simulink model "ThreeLevelANPC_16_11_22_cmv"  (R2021a)
settings: Solver=FixedStepAuto  StartTime=0.0  StopTime=0.1  RelTol=1e-3
model workspace (MAT data in the model file):
  Cdc = 0.000333333333333
  Cf = 9.4e-06
  Ctrap1 = 6e-06
  Ctrap2 = 4e-06
  DPWMGain = 1.04
  IdRef = 127
  IqRef = 0
  Lc = 0.0005
  Lf1 = 0.00015
  Lf2 = 4e-05
  Ltotal = 0.00019
  RLf1 = 0.003
  Rtrap = 0.1
  RtrapP1 = 100
  RtrapP2 = 100
  Ts = 1e-07
  Vdc = 1400
  VppRMS = 800
  fgrid = 50
  fs = 32000
  ki = 1
  ki_th = 600
  kidc = 0.1
  kidc_th = 0.05
  kp = 1
  kp_th = 600
  kpdc = 0.00166666666667
  kpdc_th = 0.05
  offset = -15
  third = 0.16
undefined symbols (not defined in the file or in its folder): C, DiscIntNeverNeededParam
libraries: spsSeriesRLCBranchLib x18, spsCurrentMeasurementLib x16, spsIGBTDiodeLib x12, spsParallelRLCBranchLib x12, spsVoltageMeasurementLib x8, spsMosfetLib x6, simulink x3, dspobslib x3, spsGroundLib x2, spsabctodq0Lib x2, eeGeneralControl x2, spsDCVoltageSourceLib x1
settings Model: OrderedModelArguments=off  Creator=ayberk.filik  LastModifiedBy=enes_
settings DataIOCC: ReturnWorkspaceOutputs=off

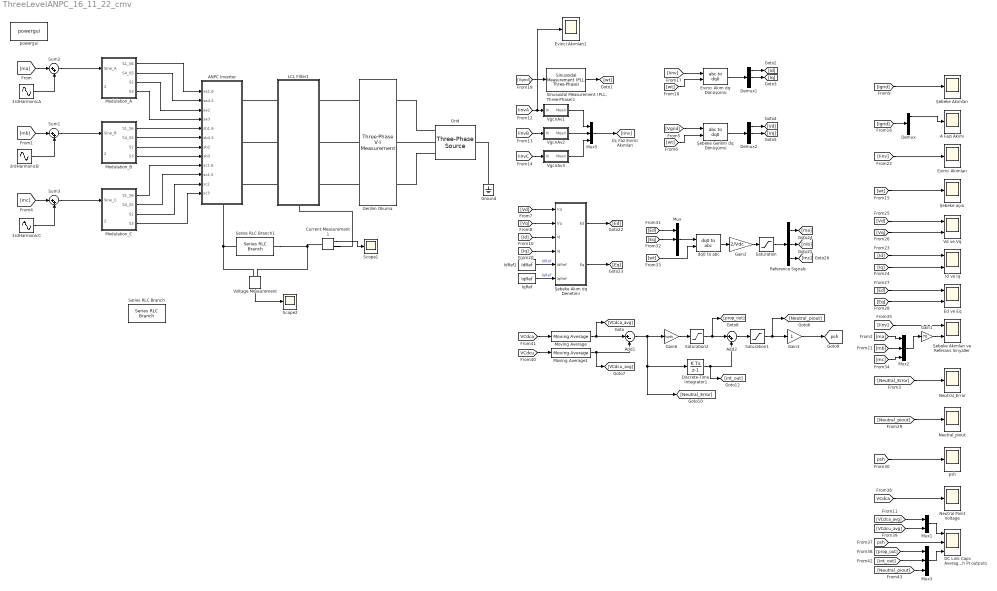
== system ThreeLevelANPC_16_11_22_cmv ==
  3rdHarmonicA : Sin  Amplitude=third  Frequency=2*pi*fgrid*3  SampleTime=0
  3rdHarmonicB : Sin  Amplitude=third  Frequency=2*pi*fgrid*3  SampleTime=0
  3rdHarmonicC : Sin  Amplitude=third  Frequency=2*pi*fgrid*3  SampleTime=0
  A Fazı Akımı : Scope
  ANPC Inverter : Subsystem
      settings: PortSchema="{\"entries\":[{\"content\":{\"sides\":[{\"content\":{\"connectorIds\":[\"In1\",\"In2\",\"In3\",\"In4\",\"In5\",\"In6\",\"In7\",\"In8\",\"In9\",\"In10\",\"In11\",\"In12\"]},\"type\":\"ConnectorPlacement.EquallySpacedRectSide\",\"uuid\":\"a224524a-50a8-4cdc-8abb-b6f444590ea5\"},{\"content\":{\"connectorIds\":[\"RConn1\",\"RConn2\",\"RConn3\"],\"side\":\"RIGHT\"},\"type\":\"ConnectorPlacement.EquallySpacedRectSide\",\"uuid\":\"5c943702-691f-470c-a624-c4353e6a6f2e\"},{\"content\":{\"connectorIds\":[],\"side\":\"TOP\"},\"type\":\"ConnectorPlacement.EquallySpacedRectSide\",\"uuid\":\"9f5f9574-c398-4dae-9e45-4c64c2b77127\"},{\"content\":{\"connectorIds\":[\"RConn4\"],\"side\":\"BOTTOM\"},\"type\":\"ConnectorPlacement.EquallySpacedRectSide\",\"uuid\":\"493948a2-9cae-4d50-8c53-e00fc1e0a563\"}]},\"type\":\"ConnectorPlacement.EquallySpacedConnector\",\"uuid\":\"1c61b5d2-4964-41af-ae3e-90cbe91c0428\"}],\"packageUris\":[\"http://schema.mathworks.com/mf0/Connector/R2020b\"],\"version\":\"1.0\"}"
  Add1 : Sum  Inputs=|+-
  Add2 : Sum  Inputs=|++
  Current Measurement1 : spsCurrentMeasurementLib/Current Measurement  PhasorSimulation=off  OutputType=Complex  PSBequivalent=0
  DC Link Caps Average Voltages psh PI outputs : Scope  NumInputPorts=3
  Demux : Demux  Outputs=3
  Demux1 : Demux  Outputs=3
  Demux2 : Demux  Outputs=3
  Discrete-Time Integrator1 : DiscreteIntegrator  gainval=kidc  SampleTime=-1  LimitOutput=on  UpperSaturationLimit=kidc_th  LowerSaturationLimit=-kidc_th  ICPrevOutput=DiscIntNeverNeededParam  ICPrevScaledInput=DiscIntNeverNeededParam
  Ed ve Eq : Scope  NumInputPorts=2
  Evirici Akım dq Dönüşümü : spsabctodq0Lib/abc to dq0  Alignment=90 degrees behind phase A axis
  Evirici Akımları : Scope
  Evirici Akımları1 : Scope
  Gain1 : Gain  Gain=70
  Gain2 : Gain  Gain=2/Vdc
  Gain3 : Gain
  Gain6 : Gain  Gain=kpdc
  Gerilim Okuma : spsThreePhaseVIMeasurementLib/Three-Phase V-I Measurement  VoltageMeasurement=phase-to-phase  SetLabelV=on  LabelV=Vgrid  Vpu=off  VpuLL=off  CurrentMeasurement=yes  SetLabelI=on  LabelI=Igrid  Ipu=off  Pbase=100e6  Vbase=500e3  OutputType=Complex  PhasorSimulation=off  PSBequivalent=0
  Grid : spsThreePhaseSourceLib/Three-Phase Source  InternalConnection=Yn  VoltagePhases=off  Voltage=VppRMS  PhaseAngle=0  Voltage_phases=[25e3 25e3 25e3]/sqrt(3)  PhaseAngles_phases=[0 -120 +120]  Frequency=fgrid  NonIdealSource=off  SpecifyImpedance=off  Resistance=0.001e-3  Inductance=0.001e-6  ShortCircuitLevel=100000e6  BaseVoltage=VppRMS  XRratio=100  BusType=swing  Pref=10e3  Qref=0  Prefabc=[10e3, 10e3, 10e3]  Qrefabc=[0, 0, 0]  Qmin=-inf  Qmax=inf
  Ground : spsGroundLib/Ground  LConnTagsString=a
  Id ve Iq : Scope  NumInputPorts=2
  IdRef1 : Constant  Value=IdRef
  IqRef : Constant  Value=IqRef
  LCL Filter1 : Subsystem
      settings: PortSchema="{\"entries\":[{\"content\":{\"sides\":[{\"content\":{\"connectorIds\":[\"LConn1\",\"LConn2\",\"LConn3\"]},\"type\":\"ConnectorPlacement.EquallySpacedRectSide\",\"uuid\":\"bea0e094-116c-4830-9da4-a9503c8d7f59\"},{\"content\":{\"connectorIds\":[\"RConn1\",\"RConn2\",\"RConn3\"],\"side\":\"RIGHT\"},\"type\":\"ConnectorPlacement.EquallySpacedRectSide\",\"uuid\":\"b52ba564-80df-4338-84ec-522ca4a71e6b\"},{\"content\":{\"connectorIds\":[],\"side\":\"TOP\"},\"type\":\"ConnectorPlacement.EquallySpacedRectSide\",\"uuid\":\"37cb4dcb-9b4f-454a-aaa0-899164a58628\"},{\"content\":{\"connectorIds\":[\"RConn4\"],\"side\":\"BOTTOM\"},\"type\":\"ConnectorPlacement.EquallySpacedRectSide\",\"uuid\":\"06a7e06c-a0ef-4b85-8c5d-00aa495f8239\"}]},\"type\":\"ConnectorPlacement.EquallySpacedConnector\",\"uuid\":\"9211e308-d4ca-451a-afa7-22bbf288c461\"}],\"packageUris\":[\"http://schema.mathworks.com/mf0/Connector/R2020b\"],\"version\":\"1.0\"}"
  Modulation_A : Subsystem
  Modulation_B : Subsystem
  Modulation_C : Subsystem
  Moving Average : eeGeneralControl/Moving Average  VariantControl=Variant1  LabelModeActiveChoice=Discrete  f=fgrid*3  x0=0  Ts=1/15000
      settings: SourceProductBaseCode=PS
  Moving Average1 : eeGeneralControl/Moving Average  VariantControl=Variant1  LabelModeActiveChoice=Discrete  f=fgrid*3  x0=0  Ts=1/15000
      settings: SourceProductBaseCode=PS
  Mux{,2..3,5} (4 alike) : Mux  Inputs=3
  Mux1 : Mux  Inputs=2
  Neutral Point Voltage : Scope
  Neutral_Error : Scope
  Neutral_piout : Scope
  Reference Signals : Demux  Outputs=3
  Saturation : Saturate  UpperLimit=1  LowerLimit=-1
  Saturation1 : Saturate  UpperLimit=0.05*2  LowerLimit=-0.05*2
  Saturation2 : Saturate  UpperLimit=kpdc_th  LowerLimit=-kpdc_th
  Scope1 : Scope
  Scope2 : Scope
  Series RLC Branch : spsSeriesRLCBranchLib/Series RLC Branch  LConnTagsString=__new0  RConnTagsString=__new0  BranchType=C  Resistance=0.001  Inductance=1e-3  SetiL0=off  InitialCurrent=0  Capacitance=100e-6  Setx0=on  InitialVoltage=0  Measurements=None
  Series RLC Branch1 : spsSeriesRLCBranchLib/Series RLC Branch  LConnTagsString=__new0  RConnTagsString=__new0  BranchType=C  Resistance=0.001  Inductance=8.0663e-03  SetiL0=off  InitialCurrent=0  Capacitance=1e-3  Setx0=on  InitialVoltage=0  Measurements=None
  "Sinusoidal Measurement (PLL, Three-Phase)1" : eeSinusoidalMeasurement/Sinusoidal Measurement (PLL, Three-Phase)  Kp_LF=150  Ki_LF=150  F0=50  Theta0=0  Ts=Ts
      settings: SourceProductBaseCode=PS
  Sum1 : Sum  Inputs=|++
  Sum2 : Sum  Inputs=|++
  Sum3 : Sum  Inputs=|++
  Vd ve Vq : Scope  NumInputPorts=2
  VgcnAv1 : Subsystem  AncestorBlock=|  DialogController=POWERSYS.PowerSysDialog  mask(Discrete Mean value){Freq=fs, Vinit=0, Ts=Ts}
      | powerlib_extras/Discrete
      | Measurements/Discrete 
      | Mean value
      mask prompts: Freq "Fundamental frequency (Hz):"; Vinit "Initial input (DC component):"; Ts "Sample time:"
      mask help: Compute the mean value of the input signal over a running window of one cycle of the specified fundamental frequency. For the first cycle of simulation, the output is held constant to the specified initial input value.
      mask init:
      | SamplesPerCycle=1/Freq/Ts;
      | RoundSamplesPerCycle=ceil(SamplesPerCycle);
      | Delay=RoundSamplesPerCycle*Ts;
      | Corr1=(SamplesPerCycle-RoundSamplesPerCycle)/2;
      | Corr2=(SamplesPerCycle-RoundSamplesPerCycle)/SamplesPerCycle;
      | K1=Corr1*Corr2;
      | K2=Corr2 + Corr1*Corr2;
      | power_initmask();
      mask Help: This block is part of a subset of blocks in the Extras library that does not have documentation associated with it, other than the block mask description.
      mask Display: disp('Mean\n(discrete)')
  VgcnAv2 : Subsystem  AncestorBlock=|  DialogController=POWERSYS.PowerSysDialog  mask(Discrete Mean value){Freq=fs, Vinit=0, Ts=Ts}
      | powerlib_extras/Discrete
      | Measurements/Discrete 
      | Mean value
      mask prompts: Freq "Fundamental frequency (Hz):"; Vinit "Initial input (DC component):"; Ts "Sample time:"
      mask help: Compute the mean value of the input signal over a running window of one cycle of the specified fundamental frequency. For the first cycle of simulation, the output is held constant to the specified initial input value.
      mask init: same as ThreeLevelANPC_16_11_22_cmv/VgcnAv1
      mask Help: This block is part of a subset of blocks in the Extras library that does not have documentation associated with it, other than the block mask description.
      mask Display: disp('Mean\n(discrete)')
  VgcnAv3 : Subsystem  AncestorBlock=|  DialogController=POWERSYS.PowerSysDialog  mask(Discrete Mean value){Freq=fs, Vinit=0, Ts=Ts}
      | powerlib_extras/Discrete
      | Measurements/Discrete 
      | Mean value
      mask prompts: Freq "Fundamental frequency (Hz):"; Vinit "Initial input (DC component):"; Ts "Sample time:"
      mask help: Compute the mean value of the input signal over a running window of one cycle of the specified fundamental frequency. For the first cycle of simulation, the output is held constant to the specified initial input value.
      mask init: same as ThreeLevelANPC_16_11_22_cmv/VgcnAv1
      mask Help: This block is part of a subset of blocks in the Extras library that does not have documentation associated with it, other than the block mask description.
      mask Display: disp('Mean\n(discrete)')
  Voltage Measurement : spsVoltageMeasurementLib/Voltage Measurement  PhasorSimulation=off  OutputType=Complex  PSBequivalent=0
  dq0 to abc : spsdq0toabcLib/dq0 to abc  Alignment=90 degrees behind phase A axis
  powergui : spspowerguiLib/powergui  Priority=1  SimulationMode=Discrete  SampleTime=Ts  frequency=60  Iterations=50  frequencyindice=0  Pbase=100e6  ErrMax=1e-4  UnitsV=kV  UnitsW=MW  buscounter=0  FunctionMessages=off  echomessages=off  EnableUseOfTLC=off  CurrentSourceSwitches=off  DisableSnubberDevices=off  DisableRonSwitches=off  DisableVfSwitches=off  DisplayEquations=off  AutomaticDiscreteSolvers=off  SolverType=Tustin/Backward Euler (TBE)  Interpol=off  ExternalGateDelay=off  methode=off  Ts=100  x0status=blocks  SPID=on  SwTol=0  HookPort=off  NonlinearTolerance=1e-4  nMaxIteration=100  ContinueOnMaxIteration=off  RestoreLinks=warning  ResistiveCurrentMeasurement=off  Frange=[0:2:500]  Ylog=off  Xlog=on  ShowGrid=off  save=off  variable=ZData  structure=0  ZoomFFT=off  StartTime=0.0  cycles=1  DisplayStyle=1  fundamental=60  FreqAxis=off  MaxFrequency=1000  frequencyindicesteady=1  RmsSteady=1  display=off
  psh : Scope
  Şebeke Akım dq Denetimi : Subsystem
  Şebeke Akımları : Scope
  Şebeke Akımları ve Referans Sinyaller : Scope  NumInputPorts=2
  Şebeke Gerilim dq Dönüşümü : spsabctodq0Lib/abc to dq0  Alignment=90 degrees behind phase A axis
  Şebeke açısı : Scope
  tag scope: psh=global
  wires:
  Modulation_A/4(S3) -> ANPC Inverter/4(sa3)
  Modulation_A/3(S2) -> ANPC Inverter/3(sa2)
  Modulation_A/2(S4_S5) -> ANPC Inverter/2(sa4,5)
  Modulation_A/1(S1_S6) -> ANPC Inverter/1(sa1,6)
  [mb] -> Sum1/1
  [mc] -> Sum3/1
  [ma] -> Sum2/1
  Mux5/1 -> [Iinv]
  [Ed] -> Mux/1
  Şebeke Akım dq Denetimi/1(Eq) -> [Eq]
  dq0 to abc/1 -> Gain2/1
  Gain2/1 -> Saturation/1
  Şebeke Akım dq Denetimi/2(Ed) -> [Ed]
  [wt] -> dq0 to abc/2
  [Eq] -> Mux/2
  Reference Signals/2 -> [mb]
  Reference Signals/3 -> [mc]
  Saturation/1 -> Reference Signals/1
  Reference Signals/1 -> [ma]
  Mux/1 -> dq0 to abc/1
  IqRef/1 -> Şebeke Akım dq Denetimi/1(IqRef)  "IqRef"
  [Vgrid] -> "Sinusoidal Measurement (PLL, Three-Phase)1"/1
  "Sinusoidal Measurement (PLL, Three-Phase)1"/2 -> [wt]
  VgcnAv1/1(Mean) -> Mux5/1
  VgcnAv2/1(Mean) -> Mux5/2
  VgcnAv3/1(Mean) -> Mux5/3
  [Igrid] -> Şebeke Akımları/1
  Modulation_B/1(S1_S6) -> ANPC Inverter/5(sb1,6)
  Modulation_B/2(S4_S5) -> ANPC Inverter/6(sb4,5)
  Modulation_B/3(S2) -> ANPC Inverter/7(sb2)
  Modulation_B/4(S3) -> ANPC Inverter/8(sb3)
  Modulation_C/4(S3) -> ANPC Inverter/12(sc3)
  Modulation_C/3(S2) -> ANPC Inverter/11(sc2)
  Modulation_C/2(S4_S5) -> ANPC Inverter/10(sc4,5)
  Modulation_C/1(S1_S6) -> ANPC Inverter/9(sc1,6)
  Sum3/1 -> Modulation_C/1(Sine_C)
  Sum1/1 -> Modulation_B/1(Sine_B)
  [IinvA] -> Evirici Akımları1/1, VgcnAv1/1(In)
  [IinvB] -> VgcnAv2/1(In)
  [IinvC] -> VgcnAv3/1(In)
  [Igrid] -> Demux/1
  Demux/1 -> A Fazı Akımı/1
  [Iinv] -> Evirici Akım dq Dönüşümü/1
  [wt] -> Evirici Akım dq Dönüşümü/2
  Evirici Akım dq Dönüşümü/1 -> Demux1/1
  Demux1/1 -> [Id]
  Demux1/2 -> [Iq]
  Demux2/2 -> [Vq]
  Demux2/1 -> [Vd]
  Şebeke Gerilim dq Dönüşümü/1 -> Demux2/1
  [wt] -> Şebeke Gerilim dq Dönüşümü/2
  [Vgrid] -> Şebeke Gerilim dq Dönüşümü/1
  [Vd] -> Şebeke Akım dq Denetimi/6(Vd)
  [Vq] -> Şebeke Akım dq Denetimi/5(Vq)
  [Id] -> Şebeke Akım dq Denetimi/4(Id)
  [Iq] -> Şebeke Akım dq Denetimi/3(Iq)
  [wt] -> Şebeke açısı/1
  [Iinv] -> Evirici Akımları/1
  [Vd] -> Vd ve Vq/1
  [Vq] -> Vd ve Vq/2
  [Id] -> Id ve Iq/1
  [Iq] -> Id ve Iq/2
  [Ed] -> Ed ve Eq/1
  [Eq] -> Ed ve Eq/2
  [Iinv] -> Şebeke Akımları ve Referans Sinyaller/1
  [mb] -> Mux2/2
  [ma] -> Mux2/1
  [mc] -> Mux2/3
  Gain1/1 -> Şebeke Akımları ve Referans Sinyaller/2
  Mux2/1 -> Gain1/1
  [Neutral_Error] -> Neutral_Error/1
  [Neutral_piout] -> Neutral_piout/1
  [psh] -> psh/1
  [VCdca] -> Neutral Point Voltage/1
  Add2/1 -> Saturation1/1
  Gain3/1 -> [psh]
  Gain6/1 -> Saturation2/1
  Discrete-Time Integrator1/1 -> [int_out], Add2/2
  [VCdca] -> Moving Average/1
  [VCdcu] -> Moving Average1/1
  Moving Average/1 -> [VCdca_avg], Add1/1
  Moving Average1/1 -> [VCdcu_avg], Add1/2
  Saturation1/1 -> [Neutral_piout], Gain3/1
  Mux1/1 -> DC Link Caps Average Voltages psh PI outputs/1
  Mux3/1 -> DC Link Caps Average Voltages psh PI outputs/3
  Saturation2/1 -> [prop_out], Add2/1
  Add1/1 -> Gain6/1, Discrete-Time Integrator1/1, [Neutral_Error]
  [VCdca_avg] -> Mux1/1
  [VCdcu_avg] -> Mux1/2
  [psh] -> DC Link Caps Average Voltages psh PI outputs/2
  [Neutral_piout] -> Mux3/3
  [int_out] -> Mux3/2
  [prop_out] -> Mux3/1
  Sum2/1 -> Modulation_A/1(Sine_A)
  3rdHarmonicA/1 -> Sum2/2
  3rdHarmonicB/1 -> Sum1/2
  3rdHarmonicC/1 -> Sum3/2
  IdRef1/1 -> Şebeke Akım dq Denetimi/2(IdRef)  "IdRef"
  Current Measurement1/1 -> Scope1/1
  Voltage Measurement/1 -> Scope2/1
  connections:
  LCL Filter1/LConn1 -- ANPC Inverter/RConn1
  LCL Filter1/LConn2 -- ANPC Inverter/RConn2
  LCL Filter1/LConn3 -- ANPC Inverter/RConn3
  Gerilim Okuma/LConn1 -- LCL Filter1/RConn1
  Gerilim Okuma/LConn2 -- LCL Filter1/RConn2
  Gerilim Okuma/LConn3 -- LCL Filter1/RConn3
  Grid/RConn2 -- Gerilim Okuma/RConn2
  Grid/RConn1 -- Gerilim Okuma/RConn1
  Grid/RConn3 -- Gerilim Okuma/RConn3
  Ground/LConn1 -- Grid/LConn1
  Voltage Measurement/LConn1 -- Current Measurement1/LConn1 -- Series RLC Branch1/LConn1
  Current Measurement1/RConn1 -- LCL Filter1/RConn4
  Voltage Measurement/LConn2 -- ANPC Inverter/RConn4 -- Series RLC Branch1/RConn1

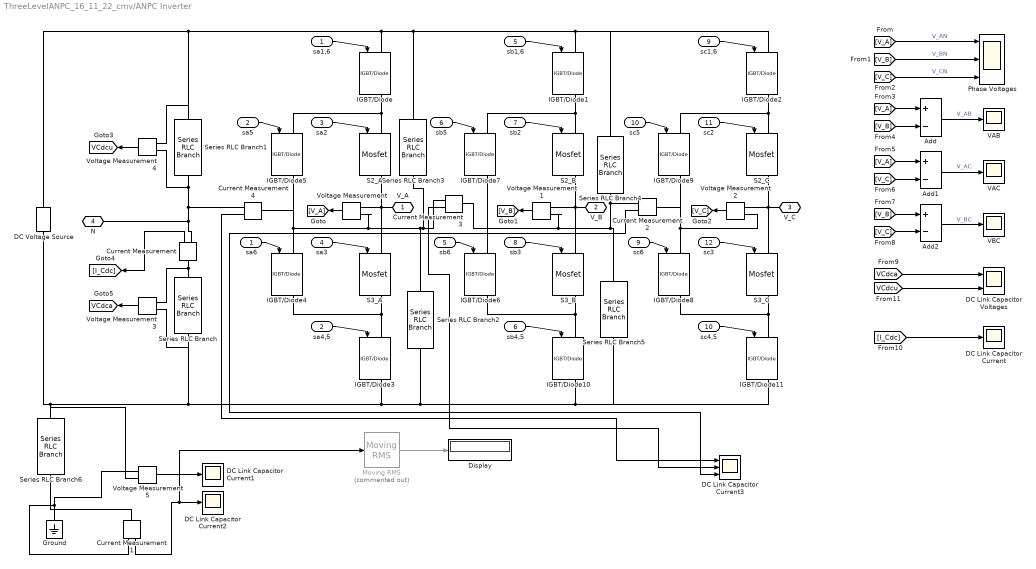
== system ThreeLevelANPC_16_11_22_cmv/ANPC Inverter ==
  sa1,6 : Inport
  sa4,5 : Inport  Port=2
  sa2 : Inport  Port=3
  sa3 : Inport  Port=4
  sb1,6 : Inport  Port=5
  sb4,5 : Inport  Port=6
  sb2 : Inport  Port=7
  sb3 : Inport  Port=8
  sc1,6 : Inport  Port=9
  sc4,5 : Inport  Port=10
  sc2 : Inport  Port=11
  sc3 : Inport  Port=12
  Add : Sum  Inputs=+-
  Add1 : Sum  Inputs=+-
  Add2 : Sum  Inputs=+-
  Current Measurement{,1..4} (5 alike) : spsCurrentMeasurementLib/Current Measurement  PhasorSimulation=off  OutputType=Complex  PSBequivalent=0
  DC Link Capacitor Current : Scope
  DC Link Capacitor Current1 : Scope
  DC Link Capacitor Current2 : Scope
  DC Link Capacitor Current3 : Scope  NumInputPorts=3
  DC Link Capacitor Voltages : Scope  NumInputPorts=2
  DC Voltage Source : spsDCVoltageSourceLib/DC Voltage Source  Amplitude=Vdc  Measurements=None
  Display : Display
  Ground : spsGroundLib/Ground  LConnTagsString=a
  IGBT/Diode{,1..11} (12 alike) : spsIGBTDiodeLib/IGBT//Diode  Ron=1e-3  Rs=1e5  Cs=inf  Measurements=on
  Moving RMS : dspstat3/Moving RMS  Commented=on  Method=Sliding window  ForgettingFactorPort=off  SpecifyWindowLength=on  WindowLength=0.02/Ts  ForgettingFactor=0.9  SimulateUsing=Code generation
      settings: SourceProductBaseCode=DS
  Phase Voltages : Scope  NumInputPorts=3
  S2_A : spsMosfetLib/Mosfet  Ron=0.1  Lon=0  Rd=0.01  Vfd=0  IC=0  Rs=1e5  Cs=inf  Measurements=on
  S2_B : spsMosfetLib/Mosfet  Ron=0.1  Lon=0  Rd=0.01  Vfd=0  IC=0  Rs=1e5  Cs=inf  Measurements=on
  S2_C : spsMosfetLib/Mosfet  Ron=0.1  Lon=0  Rd=0.01  Vfd=0  IC=0  Rs=1e5  Cs=inf  Measurements=on
  S3_A : spsMosfetLib/Mosfet  Ron=0.1  Lon=0  Rd=0.01  Vfd=0  IC=0  Rs=1e5  Cs=inf  Measurements=on
  S3_B : spsMosfetLib/Mosfet  Ron=0.1  Lon=0  Rd=0.01  Vfd=0  IC=0  Rs=1e5  Cs=inf  Measurements=on
  S3_C : spsMosfetLib/Mosfet  Ron=0.1  Lon=0  Rd=0.01  Vfd=0  IC=0  Rs=1e5  Cs=inf  Measurements=on
  Series RLC Branch{,2..5} (5 alike) : spsSeriesRLCBranchLib/Series RLC Branch  LConnTagsString=__new0  RConnTagsString=__new0  BranchType=RC  Resistance=0.001  Inductance=1e-3  SetiL0=off  InitialCurrent=0  Capacitance=Cdc/3  Setx0=on  InitialVoltage=Vdc/2-offset  Measurements=None
  Series RLC Branch1 : spsSeriesRLCBranchLib/Series RLC Branch  LConnTagsString=__new0  RConnTagsString=__new0  BranchType=RC  Resistance=0.001  Inductance=1e-3  SetiL0=off  InitialCurrent=0  Capacitance=Cdc/3  Setx0=on  InitialVoltage=Vdc/2+offset  Measurements=None
  Series RLC Branch6 : spsSeriesRLCBranchLib/Series RLC Branch  LConnTagsString=__new0  RConnTagsString=__new0  BranchType=C  Resistance=0.001  Inductance=1e-3  SetiL0=off  InitialCurrent=0  Capacitance=10e-6  Setx0=on  InitialVoltage=-Vdc/2  Measurements=None
  VAB : Scope
  VAC : Scope
  VBC : Scope
  Voltage Measurement{,1..5} (6 alike) : spsVoltageMeasurementLib/Voltage Measurement  PhasorSimulation=off  OutputType=Complex  PSBequivalent=0
  sa5 : InportShadow  Port=2
  sa6 : InportShadow
  sb5 : InportShadow  Port=6
  sb6 : InportShadow  Port=5
  sc5 : InportShadow  Port=10
  sc6 : InportShadow  Port=9
  V_A : PMIOPort  Side=Right
  V_B : PMIOPort  Port=2  Side=Right
  V_C : PMIOPort  Port=3  Side=Right
  N : PMIOPort  Port=4  Side=Right
  tag scope: VCdca=global, VCdcu=global
  wires:
  sa1,6/1 -> IGBT/Diode/1
  sa2/1 -> S2_A/1
  sa3/1 -> S3_A/1
  sa4,5/1 -> IGBT/Diode3/1
  sa6/1 -> IGBT/Diode4/1
  sa5/1 -> IGBT/Diode5/1
  sb6/1 -> IGBT/Diode6/1
  sb5/1 -> IGBT/Diode7/1
  sb3/1 -> S3_B/1
  sb2/1 -> S2_B/1
  sb1,6/1 -> IGBT/Diode1/1
  sb4,5/1 -> IGBT/Diode10/1
  Voltage Measurement/1 -> [V_A]
  Voltage Measurement1/1 -> [V_B]
  Voltage Measurement2/1 -> [V_C]
  [V_B] -> Phase Voltages/2  "V_BN"
  [V_A] -> Phase Voltages/1  "V_AN"
  [V_C] -> Phase Voltages/3  "V_CN"
  [V_A] -> Add/1
  [V_B] -> Add/2
  Add/1 -> VAB/1  "V_AB"
  Add1/1 -> VAC/1  "V_AC"
  [V_C] -> Add1/2
  [V_A] -> Add1/1
  [V_B] -> Add2/1
  [V_C] -> Add2/2
  Add2/1 -> VBC/1  "V_BC"
  sc4,5/1 -> IGBT/Diode11/1
  sc1,6/1 -> IGBT/Diode2/1
  sc2/1 -> S2_C/1
  sc3/1 -> S3_C/1
  sc5/1 -> IGBT/Diode9/1
  sc6/1 -> IGBT/Diode8/1
  Voltage Measurement3/1 -> [VCdca]
  [VCdca] -> DC Link Capacitor Voltages/1
  [I_Cdc] -> DC Link Capacitor Current/1
  Current Measurement/1 -> [I_Cdc]
  Voltage Measurement4/1 -> [VCdcu]
  [VCdcu] -> DC Link Capacitor Voltages/2
  Voltage Measurement5/1 -> DC Link Capacitor Current1/1
  Current Measurement1/1 -> Moving RMS/1, DC Link Capacitor Current2/1
  Moving RMS/1 -> Display/1
  Current Measurement2/1 -> DC Link Capacitor Current3/3
  Current Measurement3/1 -> DC Link Capacitor Current3/2
  Current Measurement4/1 -> DC Link Capacitor Current3/1
  connections:
  DC Voltage Source/RConn1 -- Voltage Measurement4/LConn1 -- Series RLC Branch1/LConn1 -- Series RLC Branch3/LConn1 -- Series RLC Branch4/LConn1 -- IGBT/Diode2/LConn1 -- IGBT/Diode1/LConn1 -- IGBT/Diode/LConn1
  IGBT/Diode3/RConn1 -- Series RLC Branch2/RConn1 -- Series RLC Branch5/RConn1 -- IGBT/Diode11/RConn1 -- IGBT/Diode10/RConn1 -- Voltage Measurement5/LConn1 -- Series RLC Branch6/LConn1 -- DC Voltage Source/LConn1 -- Voltage Measurement3/LConn2 -- Series RLC Branch/RConn1
  S2_A/LConn1 -- IGBT/Diode5/LConn1 -- IGBT/Diode/RConn1
  S2_A/RConn1 -- Voltage Measurement/LConn1 -- V_A/RConn1 -- S3_A/LConn1
  S3_A/RConn1 -- IGBT/Diode4/RConn1 -- IGBT/Diode3/LConn1
  S2_B/LConn1 -- IGBT/Diode7/LConn1 -- IGBT/Diode1/RConn1
  S3_B/RConn1 -- IGBT/Diode10/LConn1 -- IGBT/Diode6/RConn1
  S2_B/RConn1 -- Voltage Measurement1/LConn1 -- V_B/RConn1 -- S3_B/LConn1
  S2_C/LConn1 -- IGBT/Diode9/LConn1 -- IGBT/Diode2/RConn1
  S3_C/RConn1 -- IGBT/Diode11/LConn1 -- IGBT/Diode8/RConn1
  Current Measurement4/LConn1 -- IGBT/Diode5/RConn1 -- IGBT/Diode4/LConn1 -- Voltage Measurement/LConn2 -- Series RLC Branch2/LConn1 -- Current Measurement3/RConn1 -- Series RLC Branch3/RConn1
  S2_C/RConn1 -- Voltage Measurement2/LConn1 -- V_C/RConn1 -- S3_C/LConn1
  Current Measurement/LConn1 -- Voltage Measurement3/LConn1 -- Series RLC Branch/LConn1
  Voltage Measurement5/LConn2 -- Current Measurement1/RConn1 -- Ground/LConn1
  Current Measurement1/LConn1 -- Series RLC Branch6/RConn1
  IGBT/Diode8/LConn1 -- Current Measurement2/LConn1 -- IGBT/Diode9/RConn1 -- Voltage Measurement2/LConn2
  Current Measurement2/RConn1 -- Series RLC Branch5/LConn1 -- Current Measurement3/LConn1 -- IGBT/Diode7/RConn1 -- IGBT/Diode6/LConn1 -- Voltage Measurement1/LConn2 -- Series RLC Branch4/RConn1
  Voltage Measurement4/LConn2 -- Current Measurement4/RConn1 -- Current Measurement/RConn1 -- N/RConn1 -- Series RLC Branch1/RConn1

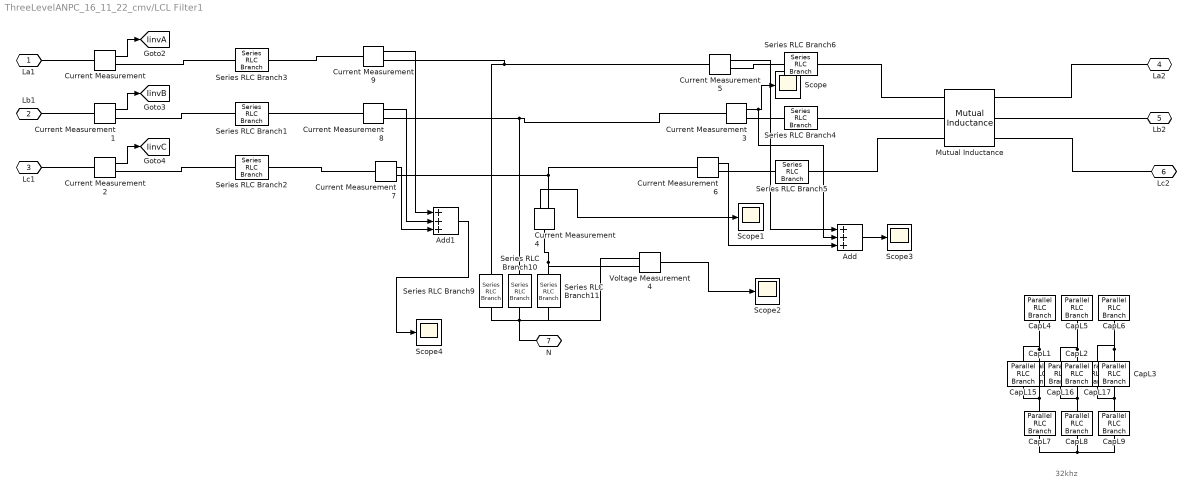
== system ThreeLevelANPC_16_11_22_cmv/LCL Filter1 ==
  note: 32khz
  Add : Sum  Inputs=+++
  Add1 : Sum  Inputs=+++
  CapL1 : spsParallelRLCBranchLib/Parallel RLC Branch  LConnTagsString=a  RConnTagsString=__new0  BranchType=L  Resistance=1  Inductance=1/(4*pi^2*(1*fs)^2*Ctrap1)  SetiL0=off  InitialCurrent=0  Capacitance=C  Setx0=off  InitialVoltage=0  Measurements=None
  CapL15 : spsParallelRLCBranchLib/Parallel RLC Branch  LConnTagsString=a  RConnTagsString=__new0  BranchType=R  Resistance=RtrapP2  Inductance=12.655e-6  SetiL0=off  InitialCurrent=0  Capacitance=C  Setx0=off  InitialVoltage=0  Measurements=None
  CapL16 : spsParallelRLCBranchLib/Parallel RLC Branch  LConnTagsString=a  RConnTagsString=__new0  BranchType=R  Resistance=RtrapP2  Inductance=12.655e-6  SetiL0=off  InitialCurrent=0  Capacitance=C  Setx0=off  InitialVoltage=0  Measurements=None
  CapL17 : spsParallelRLCBranchLib/Parallel RLC Branch  LConnTagsString=a  RConnTagsString=__new0  BranchType=R  Resistance=RtrapP2  Inductance=12.655e-6  SetiL0=off  InitialCurrent=0  Capacitance=C  Setx0=off  InitialVoltage=0  Measurements=None
  CapL2 : spsParallelRLCBranchLib/Parallel RLC Branch  LConnTagsString=a  RConnTagsString=__new0  BranchType=L  Resistance=1  Inductance=1/(4*pi^2*(1*fs)^2*Ctrap1)  SetiL0=off  InitialCurrent=0  Capacitance=C  Setx0=off  InitialVoltage=-250  Measurements=None
  CapL3 : spsParallelRLCBranchLib/Parallel RLC Branch  LConnTagsString=a  RConnTagsString=__new0  BranchType=L  Resistance=1  Inductance=1/(4*pi^2*(1*fs)^2*Ctrap1)  SetiL0=off  InitialCurrent=0  Capacitance=C  Setx0=off  InitialVoltage=250  Measurements=None
  CapL4 : spsParallelRLCBranchLib/Parallel RLC Branch  LConnTagsString=a  RConnTagsString=__new0  BranchType=R  Resistance=Rtrap  Inductance=12.655e-6  SetiL0=off  InitialCurrent=0  Capacitance=C  Setx0=off  InitialVoltage=0  Measurements=None
  CapL5 : spsParallelRLCBranchLib/Parallel RLC Branch  LConnTagsString=a  RConnTagsString=__new0  BranchType=R  Resistance=Rtrap  Inductance=0.1  SetiL0=off  InitialCurrent=0  Capacitance=C  Setx0=off  InitialVoltage=-250  Measurements=None
  CapL6 : spsParallelRLCBranchLib/Parallel RLC Branch  LConnTagsString=a  RConnTagsString=__new0  BranchType=R  Resistance=Rtrap  Inductance=0.1  SetiL0=off  InitialCurrent=0  Capacitance=C  Setx0=off  InitialVoltage=250  Measurements=None
  CapL7 : spsParallelRLCBranchLib/Parallel RLC Branch  LConnTagsString=a  RConnTagsString=__new0  BranchType=C  Resistance=1  Inductance=1e-3  SetiL0=off  InitialCurrent=0  Capacitance=Ctrap1  Setx0=off  InitialVoltage=0  Measurements=None
  CapL8 : spsParallelRLCBranchLib/Parallel RLC Branch  LConnTagsString=a  RConnTagsString=__new0  BranchType=C  Resistance=1  Inductance=1e-3  SetiL0=off  InitialCurrent=0  Capacitance=Ctrap1  Setx0=off  InitialVoltage=-250  Measurements=None
  CapL9 : spsParallelRLCBranchLib/Parallel RLC Branch  LConnTagsString=a  RConnTagsString=__new0  BranchType=C  Resistance=1  Inductance=1e-3  SetiL0=off  InitialCurrent=0  Capacitance=Ctrap1  Setx0=off  InitialVoltage=250  Measurements=None
  Current Measurement{,1..9} (10 alike) : spsCurrentMeasurementLib/Current Measurement  PhasorSimulation=off  OutputType=Complex  PSBequivalent=0
  Mutual Inductance : spsMutualInductanceLib/Mutual Inductance  LConnTagsString=a|b|c  RConnTagsString=A|B|C  TypeOfMutual=Generalized mutual inductance  NumberOfWindings=3  SelfImpedance1=[1.1 1.1e-03]  SelfImpedance2=[ 1.1 1.1e-03]  ThreeWindings=on  SelfImpedance3=[ 1.1 1.1e-03]  MutualImpedance=[1.0 1.0e-03]  InductanceMatrix="[1.0 0.95  0.95 ;  0.95 1.0  0.95;  0.95 0.95 1.0 ] * Lc"  ResistanceMatrix="[1.0 0.9  0.9 ;  0.9 1.0  0.9;  0.9 0.9 1.0 ] *10"  Measurements=None
      settings: SourceProductBaseCode=PS
  Scope{,1..4} (5 alike) : Scope
  Series RLC Branch1 : spsSeriesRLCBranchLib/Series RLC Branch  LConnTagsString=__new0  RConnTagsString=__new0  BranchType=RL  Resistance=RLf1  Inductance=Lf1  SetiL0=off  InitialCurrent=-60  Capacitance=1e-6  Setx0=off  InitialVoltage=0  Measurements=None
  Series RLC Branch10 : spsSeriesRLCBranchLib/Series RLC Branch  LConnTagsString=__new0  RConnTagsString=__new0  BranchType=RC  Resistance=0.0042  Inductance=0.2e-3  SetiL0=off  InitialCurrent=0  Capacitance=Cf  Setx0=off  InitialVoltage=0  Measurements=None
  Series RLC Branch11 : spsSeriesRLCBranchLib/Series RLC Branch  LConnTagsString=__new0  RConnTagsString=__new0  BranchType=RC  Resistance=0.0042  Inductance=0.2e-3  SetiL0=off  InitialCurrent=0  Capacitance=Cf  Setx0=off  InitialVoltage=0  Measurements=None
  Series RLC Branch2 : spsSeriesRLCBranchLib/Series RLC Branch  LConnTagsString=__new0  RConnTagsString=__new0  BranchType=RL  Resistance=RLf1  Inductance=Lf1  SetiL0=off  InitialCurrent=60  Capacitance=1e-6  Setx0=off  InitialVoltage=0  Measurements=None
  Series RLC Branch3 : spsSeriesRLCBranchLib/Series RLC Branch  LConnTagsString=__new0  RConnTagsString=__new0  BranchType=RL  Resistance=RLf1  Inductance=Lf1  SetiL0=off  InitialCurrent=0  Capacitance=1e-6  Setx0=off  InitialVoltage=0  Measurements=None
  Series RLC Branch4 : spsSeriesRLCBranchLib/Series RLC Branch  LConnTagsString=__new0  RConnTagsString=__new0  BranchType=RL  Resistance=0.001  Inductance=Lf2  SetiL0=off  InitialCurrent=-60  Capacitance=1e-6  Setx0=off  InitialVoltage=0  Measurements=None
  Series RLC Branch5 : spsSeriesRLCBranchLib/Series RLC Branch  LConnTagsString=__new0  RConnTagsString=__new0  BranchType=RL  Resistance=0.001  Inductance=Lf2  SetiL0=off  InitialCurrent=60  Capacitance=1e-6  Setx0=off  InitialVoltage=0  Measurements=None
  Series RLC Branch6 : spsSeriesRLCBranchLib/Series RLC Branch  LConnTagsString=__new0  RConnTagsString=__new0  BranchType=RL  Resistance=0.001  Inductance=Lf2  SetiL0=off  InitialCurrent=0  Capacitance=1e-6  Setx0=off  InitialVoltage=0  Measurements=None
  Series RLC Branch9 : spsSeriesRLCBranchLib/Series RLC Branch  LConnTagsString=__new0  RConnTagsString=__new0  BranchType=RC  Resistance=0.0042  Inductance=0.2e-3  SetiL0=off  InitialCurrent=0  Capacitance=Cf  Setx0=off  InitialVoltage=0  Measurements=None
  Voltage Measurement4 : spsVoltageMeasurementLib/Voltage Measurement  PhasorSimulation=off  OutputType=Complex  PSBequivalent=0
  La1 : PMIOPort  Side=Left
  Lb1 : PMIOPort  Port=2  Side=Left
  Lc1 : PMIOPort  Port=3  Side=Left
  La2 : PMIOPort  Port=4  Side=Right
  Lb2 : PMIOPort  Port=5  Side=Right
  Lc2 : PMIOPort  Port=6  Side=Right
  N : PMIOPort  Port=7  Side=Right
  tag scope: IinvA=global, IinvB=global, IinvC=global
  wires:
  Current Measurement/1 -> [IinvA]
  Current Measurement1/1 -> [IinvB]
  Current Measurement2/1 -> [IinvC]
  Current Measurement3/1 -> Add/2, Scope/1
  Current Measurement4/1 -> Scope1/1
  Voltage Measurement4/1 -> Scope2/1
  Current Measurement5/1 -> Add/1
  Current Measurement6/1 -> Add/3
  Add/1 -> Scope3/1
  Current Measurement9/1 -> Add1/1
  Current Measurement8/1 -> Add1/2
  Current Measurement7/1 -> Add1/3
  Add1/1 -> Scope4/1
  connections:
  Series RLC Branch10/RConn1 -- Voltage Measurement4/LConn2 -- Series RLC Branch11/RConn1 -- N/RConn1 -- Series RLC Branch9/RConn1
  Series RLC Branch3/LConn1 -- Current Measurement/RConn1
  Current Measurement6/LConn1 -- Current Measurement7/RConn1 -- Current Measurement4/RConn1
  Series RLC Branch9/LConn1 -- Current Measurement9/RConn1 -- Current Measurement5/LConn1
  Current Measurement3/LConn1 -- Current Measurement8/RConn1 -- Series RLC Branch10/LConn1
  CapL3/RConn1 -- CapL9/LConn1 -- CapL17/RConn1
  CapL2/RConn1 -- CapL8/LConn1 -- CapL16/RConn1
  CapL2/LConn1 -- CapL5/RConn1 -- CapL16/LConn1
  CapL3/LConn1 -- CapL6/RConn1 -- CapL17/LConn1
  CapL1/RConn1 -- CapL7/LConn1 -- CapL15/RConn1
  CapL7/RConn1 -- CapL8/RConn1 -- CapL9/RConn1
  CapL1/LConn1 -- CapL4/RConn1 -- CapL15/LConn1
  Current Measurement1/LConn1 -- Lb1/RConn1
  Current Measurement1/RConn1 -- Series RLC Branch1/LConn1
  Current Measurement2/RConn1 -- Series RLC Branch2/LConn1
  Current Measurement/LConn1 -- La1/RConn1
  Current Measurement2/LConn1 -- Lc1/RConn1
  Current Measurement3/RConn1 -- Series RLC Branch4/LConn1
  Current Measurement4/LConn1 -- Voltage Measurement4/LConn1 -- Series RLC Branch11/LConn1
  Mutual Inductance/LConn2 -- Series RLC Branch4/RConn1
  Mutual Inductance/RConn2 -- Lb2/RConn1
  Series RLC Branch5/RConn1 -- Mutual Inductance/LConn3
  Mutual Inductance/RConn3 -- Lc2/RConn1
  Series RLC Branch6/RConn1 -- Mutual Inductance/LConn1
  Mutual Inductance/RConn1 -- La2/RConn1
  Current Measurement5/RConn1 -- Series RLC Branch6/LConn1
  Current Measurement6/RConn1 -- Series RLC Branch5/LConn1
  Series RLC Branch3/RConn1 -- Current Measurement9/LConn1
  Series RLC Branch1/RConn1 -- Current Measurement8/LConn1
  Series RLC Branch2/RConn1 -- Current Measurement7/LConn1

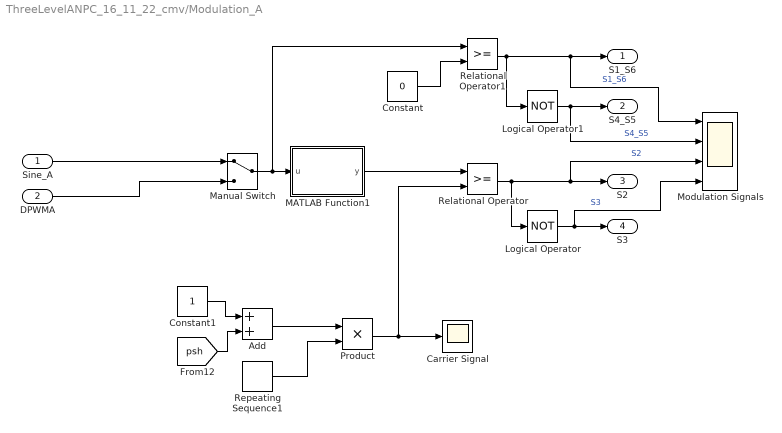
== system ThreeLevelANPC_16_11_22_cmv/Modulation_A ==
  Sine_A : Inport
  DPWMA : Inport  Port=2
  Add : Sum
  Carrier Signal : Scope
  Constant : Constant  Value=0
  Constant1 : Constant
  Logical Operator : Logic  Operator=NOT  AllPortsSameDT=off  OutDataTypeStr=boolean
  Logical Operator1 : Logic  Operator=NOT  AllPortsSameDT=off  OutDataTypeStr=boolean
  MATLAB Function1 : MATLAB Function  TreatAsAtomicUnit=on
  Manual Switch : ManualSwitch
  Modulation Signals : Scope  NumInputPorts=4
  Product : Product
  Relational Operator : RelationalOperator  OutDataTypeStr=boolean  RndMeth=Simplest
  Relational Operator1 : RelationalOperator  OutDataTypeStr=boolean  RndMeth=Simplest
  Repeating Sequence1 : simulink/Sources/Repeating Sequence  rep_seq_t=[0 0.5/fs 1/fs]  rep_seq_y=[0 (1) 0]
  S1_S6 : Outport
  S4_S5 : Outport  Port=2
  S2 : Outport  Port=3
  S3 : Outport  Port=4
  wires:
  Relational Operator/1 -> Logical Operator/1, S2/1, Modulation Signals/3  "S2"
  Relational Operator1/1 -> Logical Operator1/1, S1_S6/1, Modulation Signals/1  "S1_S6"
  Logical Operator/1 -> S3/1, Modulation Signals/4  "S3"
  Constant/1 -> Relational Operator1/2
  Logical Operator1/1 -> S4_S5/1, Modulation Signals/2  "S4_S5"
  MATLAB Function1/1(y) -> Relational Operator/1
  Sine_A/1 -> Manual Switch/1
  Manual Switch/1 -> Relational Operator1/1, MATLAB Function1/1(u)
  Constant1/1 -> Add/1
  [psh] -> Add/2
  Add/1 -> Product/1
  Repeating Sequence1/1 -> Product/2
  Product/1 -> Carrier Signal/1, Relational Operator/2
  DPWMA/1 -> Manual Switch/2

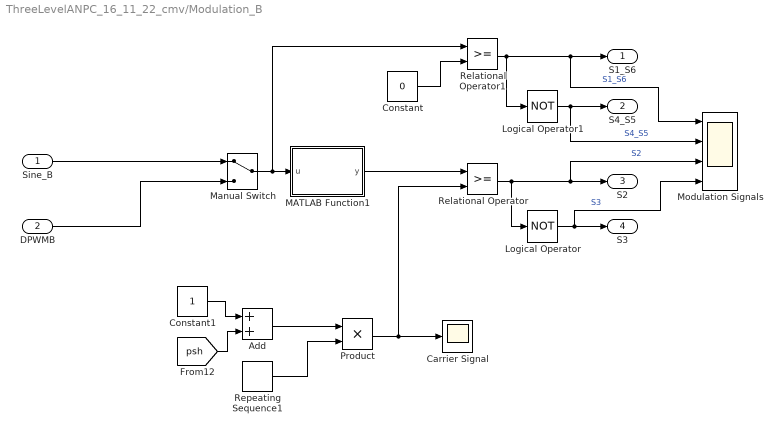
== system ThreeLevelANPC_16_11_22_cmv/Modulation_B ==
  Sine_B : Inport
  DPWMB : Inport  Port=2
  Add : Sum
  Carrier Signal : Scope
  Constant : Constant  Value=0
  Constant1 : Constant
  Logical Operator : Logic  Operator=NOT  AllPortsSameDT=off  OutDataTypeStr=boolean
  Logical Operator1 : Logic  Operator=NOT  AllPortsSameDT=off  OutDataTypeStr=boolean
  MATLAB Function1 : MATLAB Function  TreatAsAtomicUnit=on
  Manual Switch : ManualSwitch
  Modulation Signals : Scope  NumInputPorts=4
  Product : Product
  Relational Operator : RelationalOperator  OutDataTypeStr=boolean  RndMeth=Simplest
  Relational Operator1 : RelationalOperator  OutDataTypeStr=boolean  RndMeth=Simplest
  Repeating Sequence1 : simulink/Sources/Repeating Sequence  rep_seq_t=[0 0.5/fs 1/fs]  rep_seq_y=[0 (1) 0]
  S1_S6 : Outport
  S4_S5 : Outport  Port=2
  S2 : Outport  Port=3
  S3 : Outport  Port=4
  wires:
  DPWMB/1 -> Manual Switch/2
  Add/1 -> Product/1
  Logical Operator/1 -> S3/1, Modulation Signals/4  "S3"
  Manual Switch/1 -> Relational Operator1/1, MATLAB Function1/1(u)
  Repeating Sequence1/1 -> Product/2
  [psh] -> Add/2
  Constant1/1 -> Add/1
  Product/1 -> Carrier Signal/1, Relational Operator/2
  Logical Operator1/1 -> S4_S5/1, Modulation Signals/2  "S4_S5"
  Sine_B/1 -> Manual Switch/1
  Relational Operator1/1 -> Logical Operator1/1, S1_S6/1, Modulation Signals/1  "S1_S6"
  Relational Operator/1 -> Logical Operator/1, S2/1, Modulation Signals/3  "S2"
  MATLAB Function1/1(y) -> Relational Operator/1
  Constant/1 -> Relational Operator1/2

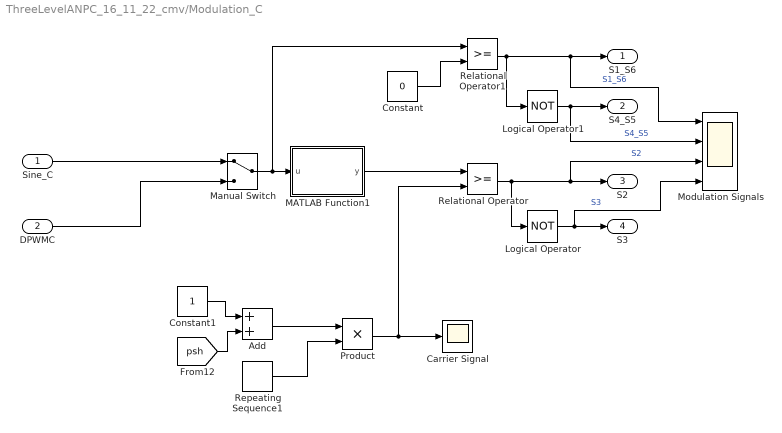
== system ThreeLevelANPC_16_11_22_cmv/Modulation_C ==
  Sine_C : Inport
  DPWMC : Inport  Port=2
  Add : Sum
  Carrier Signal : Scope
  Constant : Constant  Value=0
  Constant1 : Constant
  Logical Operator : Logic  Operator=NOT  AllPortsSameDT=off  OutDataTypeStr=boolean
  Logical Operator1 : Logic  Operator=NOT  AllPortsSameDT=off  OutDataTypeStr=boolean
  MATLAB Function1 : MATLAB Function  TreatAsAtomicUnit=on
  Manual Switch : ManualSwitch
  Modulation Signals : Scope  NumInputPorts=4
  Product : Product
  Relational Operator : RelationalOperator  OutDataTypeStr=boolean  RndMeth=Simplest
  Relational Operator1 : RelationalOperator  OutDataTypeStr=boolean  RndMeth=Simplest
  Repeating Sequence1 : simulink/Sources/Repeating Sequence  rep_seq_t=[0 0.5/fs 1/fs]  rep_seq_y=[0 (1) 0]
  S1_S6 : Outport
  S4_S5 : Outport  Port=2
  S2 : Outport  Port=3
  S3 : Outport  Port=4
  wires:
  DPWMC/1 -> Manual Switch/2
  Add/1 -> Product/1
  Logical Operator/1 -> S3/1, Modulation Signals/4  "S3"
  Manual Switch/1 -> Relational Operator1/1, MATLAB Function1/1(u)
  Repeating Sequence1/1 -> Product/2
  [psh] -> Add/2
  Constant1/1 -> Add/1
  Product/1 -> Carrier Signal/1, Relational Operator/2
  Logical Operator1/1 -> S4_S5/1, Modulation Signals/2  "S4_S5"
  Sine_C/1 -> Manual Switch/1
  Relational Operator1/1 -> Logical Operator1/1, S1_S6/1, Modulation Signals/1  "S1_S6"
  Relational Operator/1 -> Logical Operator/1, S2/1, Modulation Signals/3  "S2"
  MATLAB Function1/1(y) -> Relational Operator/1
  Constant/1 -> Relational Operator1/2

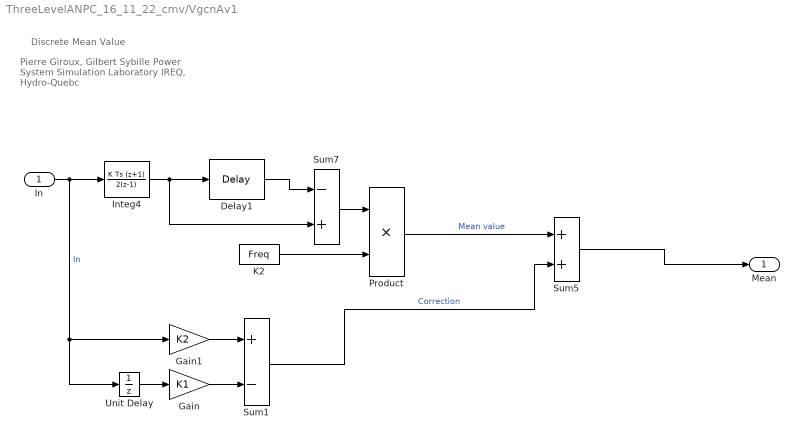
== system ThreeLevelANPC_16_11_22_cmv/VgcnAv1 ==
  note: Discrete Mean Value
  note: Pierre Giroux, Gilbert Sybille
      | Power System Simulation Laboratory
      | IREQ, Hydro-Quebc
  In : Inport
  Delay1 : dspobslib/Delay  InputProcessing=Columns as channels (frame based)  dly_unit=Samples  delay=round(1/(fs*Ts))  ic_detail=off  dif_ic_for_ch=off  dif_ic_for_dly=off  ic=0  reset_popup=None
      settings: SourceProductBaseCode=DS
  Gain : Gain  Gain=K1  SaturateOnIntegerOverflow=on  OutDataTypeStr=Inherit: Same as input  ParamDataTypeStr=Inherit: Same as input
  Gain1 : Gain  Gain=K2  SaturateOnIntegerOverflow=on  OutDataTypeStr=Inherit: Same as input  ParamDataTypeStr=Inherit: Same as input
  Integ4 : DiscreteIntegrator  IntegratorMethod=Integration: Trapezoidal  SampleTime=Ts  ICPrevOutput=DiscIntNeverNeededParam  ICPrevScaledInput=DiscIntNeverNeededParam
  K2 : Constant  Value=Freq  SampleTime=Ts
  Product : Product  InputSameDT=on  SaturateOnIntegerOverflow=on  OutDataTypeStr=Inherit: Same as first input
  Sum1 : Sum  Inputs=+-  InputSameDT=on  SaturateOnIntegerOverflow=on  OutDataTypeStr=Inherit: Same as first input
  Sum5 : Sum  InputSameDT=on  SaturateOnIntegerOverflow=on  OutDataTypeStr=Inherit: Same as first input
  Sum7 : Sum  Inputs=-+  InputSameDT=on  SaturateOnIntegerOverflow=on  OutDataTypeStr=Inherit: Same as first input
  Unit Delay : UnitDelay  SampleTime=Ts  HasFrameUpgradeWarning=on
  Mean : Outport  VectorParamsAs1DForOutWhenUnconnected=off
  wires:
  Delay1/1 -> Sum7/1
  Sum1/1 -> Sum5/2  "Correction"
  Gain/1 -> Sum1/2
  Unit Delay/1 -> Gain/1
  Gain1/1 -> Sum1/1
  Sum5/1 -> Mean/1
  In/1 -> Unit Delay/1, Gain1/1, Integ4/1  "In"
  K2/1 -> Product/2
  Integ4/1 -> Sum7/2, Delay1/1
  Sum7/1 -> Product/1
  Product/1 -> Sum5/1  "Mean value"

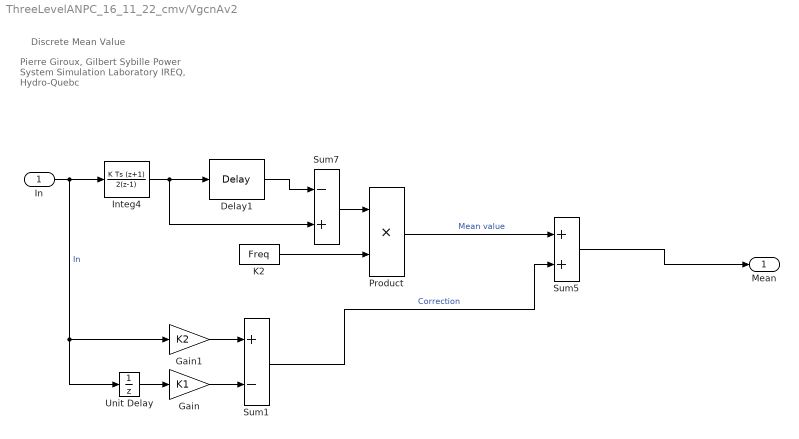
== system ThreeLevelANPC_16_11_22_cmv/VgcnAv2 ==
  note: Discrete Mean Value
  note: Pierre Giroux, Gilbert Sybille
      | Power System Simulation Laboratory
      | IREQ, Hydro-Quebc
  In : Inport
  Delay1 : dspobslib/Delay  InputProcessing=Columns as channels (frame based)  dly_unit=Samples  delay=round(1/(fs*Ts))  ic_detail=off  dif_ic_for_ch=off  dif_ic_for_dly=off  ic=0  reset_popup=None
      settings: SourceProductBaseCode=DS
  Gain : Gain  Gain=K1  SaturateOnIntegerOverflow=on  OutDataTypeStr=Inherit: Same as input  ParamDataTypeStr=Inherit: Same as input
  Gain1 : Gain  Gain=K2  SaturateOnIntegerOverflow=on  OutDataTypeStr=Inherit: Same as input  ParamDataTypeStr=Inherit: Same as input
  Integ4 : DiscreteIntegrator  IntegratorMethod=Integration: Trapezoidal  SampleTime=Ts  ICPrevOutput=DiscIntNeverNeededParam  ICPrevScaledInput=DiscIntNeverNeededParam
  K2 : Constant  Value=Freq  SampleTime=Ts
  Product : Product  InputSameDT=on  SaturateOnIntegerOverflow=on  OutDataTypeStr=Inherit: Same as first input
  Sum1 : Sum  Inputs=+-  InputSameDT=on  SaturateOnIntegerOverflow=on  OutDataTypeStr=Inherit: Same as first input
  Sum5 : Sum  InputSameDT=on  SaturateOnIntegerOverflow=on  OutDataTypeStr=Inherit: Same as first input
  Sum7 : Sum  Inputs=-+  InputSameDT=on  SaturateOnIntegerOverflow=on  OutDataTypeStr=Inherit: Same as first input
  Unit Delay : UnitDelay  SampleTime=Ts  HasFrameUpgradeWarning=on
  Mean : Outport  VectorParamsAs1DForOutWhenUnconnected=off
  wires:
  Delay1/1 -> Sum7/1
  Sum1/1 -> Sum5/2  "Correction"
  Gain/1 -> Sum1/2
  Unit Delay/1 -> Gain/1
  Gain1/1 -> Sum1/1
  Sum5/1 -> Mean/1
  In/1 -> Unit Delay/1, Gain1/1, Integ4/1  "In"
  K2/1 -> Product/2
  Integ4/1 -> Sum7/2, Delay1/1
  Sum7/1 -> Product/1
  Product/1 -> Sum5/1  "Mean value"

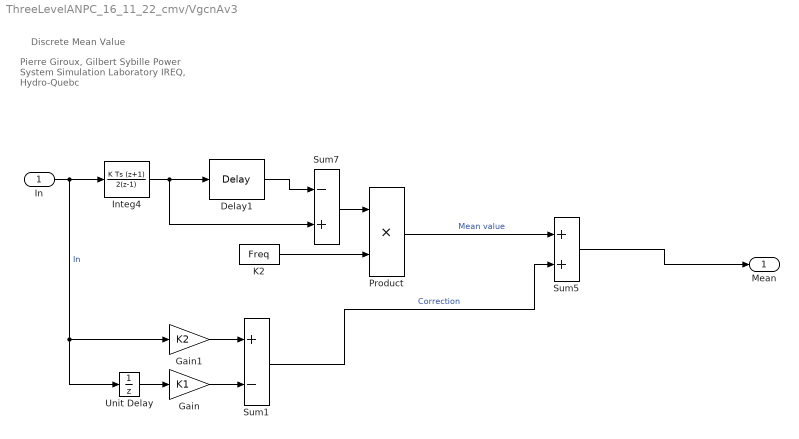
== system ThreeLevelANPC_16_11_22_cmv/VgcnAv3 ==
  note: Discrete Mean Value
  note: Pierre Giroux, Gilbert Sybille
      | Power System Simulation Laboratory
      | IREQ, Hydro-Quebc
  In : Inport
  Delay1 : dspobslib/Delay  InputProcessing=Columns as channels (frame based)  dly_unit=Samples  delay=round(1/(fs*Ts))  ic_detail=off  dif_ic_for_ch=off  dif_ic_for_dly=off  ic=0  reset_popup=None
      settings: SourceProductBaseCode=DS
  Gain : Gain  Gain=K1  SaturateOnIntegerOverflow=on  OutDataTypeStr=Inherit: Same as input  ParamDataTypeStr=Inherit: Same as input
  Gain1 : Gain  Gain=K2  SaturateOnIntegerOverflow=on  OutDataTypeStr=Inherit: Same as input  ParamDataTypeStr=Inherit: Same as input
  Integ4 : DiscreteIntegrator  IntegratorMethod=Integration: Trapezoidal  SampleTime=Ts  ICPrevOutput=DiscIntNeverNeededParam  ICPrevScaledInput=DiscIntNeverNeededParam
  K2 : Constant  Value=Freq  SampleTime=Ts
  Product : Product  InputSameDT=on  SaturateOnIntegerOverflow=on  OutDataTypeStr=Inherit: Same as first input
  Sum1 : Sum  Inputs=+-  InputSameDT=on  SaturateOnIntegerOverflow=on  OutDataTypeStr=Inherit: Same as first input
  Sum5 : Sum  InputSameDT=on  SaturateOnIntegerOverflow=on  OutDataTypeStr=Inherit: Same as first input
  Sum7 : Sum  Inputs=-+  InputSameDT=on  SaturateOnIntegerOverflow=on  OutDataTypeStr=Inherit: Same as first input
  Unit Delay : UnitDelay  SampleTime=Ts  HasFrameUpgradeWarning=on
  Mean : Outport  VectorParamsAs1DForOutWhenUnconnected=off
  wires:
  Delay1/1 -> Sum7/1
  Sum1/1 -> Sum5/2  "Correction"
  Gain/1 -> Sum1/2
  Unit Delay/1 -> Gain/1
  Gain1/1 -> Sum1/1
  Sum5/1 -> Mean/1
  In/1 -> Unit Delay/1, Gain1/1, Integ4/1  "In"
  K2/1 -> Product/2
  Integ4/1 -> Sum7/2, Delay1/1
  Sum7/1 -> Product/1
  Product/1 -> Sum5/1  "Mean value"

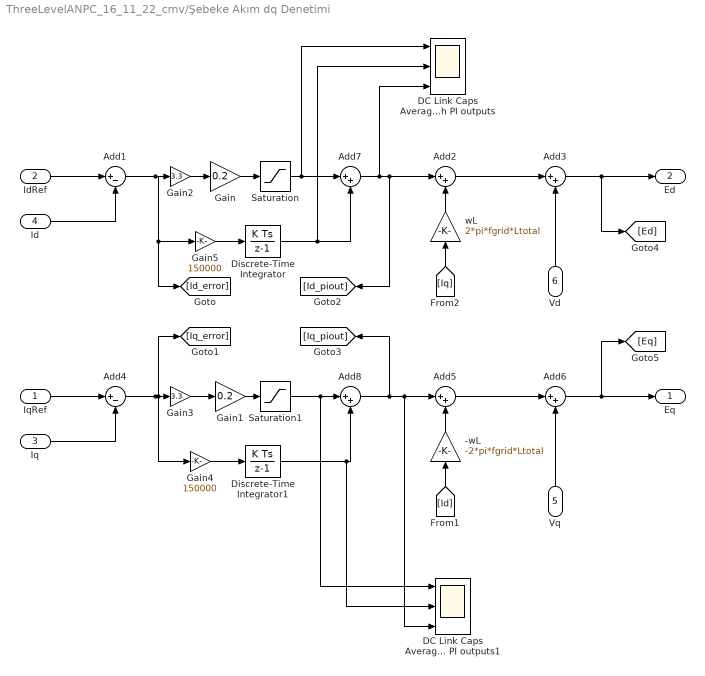
== system ThreeLevelANPC_16_11_22_cmv/Şebeke Akım dq Denetimi ==
  IqRef : Inport
  IdRef : Inport  Port=2
  Iq : Inport  Port=3
  Id : Inport  Port=4
  Vq : Inport  Port=5
  Vd : Inport  Port=6
  -wL : Gain  Gain=-2*pi*fgrid*Ltotal
  Add1 : Sum  Inputs=|+-
  Add{2..3,5..8} (6 alike) : Sum  Inputs=|++
  Add4 : Sum  Inputs=|+-
  DC Link Caps Average Voltages psh PI outputs : Scope  NumInputPorts=3
  DC Link Caps Average Voltages psh PI outputs1 : Scope  NumInputPorts=3
  Discrete-Time Integrator : DiscreteIntegrator  gainval=ki  InitialCondition=-525  SampleTime=-1  LimitOutput=on  UpperSaturationLimit=ki_th  LowerSaturationLimit=-ki_th  ICPrevOutput=DiscIntNeverNeededParam  ICPrevScaledInput=DiscIntNeverNeededParam
  Discrete-Time Integrator1 : DiscreteIntegrator  gainval=ki  InitialCondition=-330  SampleTime=-1  LimitOutput=on  UpperSaturationLimit=ki_th  LowerSaturationLimit=-ki_th  ICPrevOutput=DiscIntNeverNeededParam  ICPrevScaledInput=DiscIntNeverNeededParam
  Gain : Gain  Gain=0.2
  Gain1 : Gain  Gain=0.2
  Gain2 : Gain  Gain=3.3
  Gain3 : Gain  Gain=3.3
  Gain4 : Gain  Gain=150000
  Gain5 : Gain  Gain=150000
  Saturation : Saturate  UpperLimit=kp_th  LowerLimit=-kp_th
  Saturation1 : Saturate  UpperLimit=kp_th  LowerLimit=-kp_th
  wL : Gain  Gain=2*pi*fgrid*Ltotal
  Eq : Outport
  Ed : Outport  Port=2
  wires:
  Add1/1 -> [Id_error], Gain5/1, Gain2/1
  Vd/1 -> Add3/2
  wL/1 -> Add2/2
  Add2/1 -> Add3/1
  Add3/1 -> [Ed], Ed/1
  [Iq] -> wL/1
  Id/1 -> Add1/2
  IdRef/1 -> Add1/1
  Gain/1 -> Saturation/1
  Saturation/1 -> DC Link Caps Average Voltages psh PI outputs/1, Add7/1
  Discrete-Time Integrator/1 -> DC Link Caps Average Voltages psh PI outputs/2, Add7/2
  Add7/1 -> DC Link Caps Average Voltages psh PI outputs/3, [Id_piout], Add2/1
  Add8/1 -> [Iq_piout], DC Link Caps Average Voltages psh PI outputs1/3, Add5/1
  Discrete-Time Integrator1/1 -> DC Link Caps Average Voltages psh PI outputs1/2, Add8/2
  Saturation1/1 -> DC Link Caps Average Voltages psh PI outputs1/1, Add8/1
  Gain1/1 -> Saturation1/1
  IqRef/1 -> Add4/1
  Iq/1 -> Add4/2
  [Id] -> -wL/1
  Add6/1 -> [Eq], Eq/1
  Add5/1 -> Add6/1
  -wL/1 -> Add5/2
  Vq/1 -> Add6/2
  Add4/1 -> Gain4/1, [Iq_error], Gain3/1
  Gain2/1 -> Gain/1
  Gain3/1 -> Gain1/1
  Gain4/1 -> Discrete-Time Integrator1/1
  Gain5/1 -> Discrete-Time Integrator/1

== matlab function ThreeLevelANPC_16_11_22_cmv/Modulation_C/MATLAB Function1 ==
  data: u input; y output
function y = fcn(u)

ma = 1;

if u >= 0
    y = u;
else
    y = u + ma;
end

== matlab function ThreeLevelANPC_16_11_22_cmv/Modulation_A/MATLAB Function1 ==
  data: u input; y output
function y = fcn(u)

ma = 1;

if u >= 0
    y = u;
else
    y = u + ma;
end

== matlab function ThreeLevelANPC_16_11_22_cmv/Modulation_B/MATLAB Function1 ==
  data: u input; y output
function y = fcn(u)

ma = 1;

if u >= 0
    y = u;
else
    y = u + ma;
end
